simulink model "SquareRootEstimation"  (R2022b)
settings: Solver=ode23  StartTime=0.0  StopTime=10  RelTol=1e-7  AbsTol=1e-7
settings Model: Creator=aless  LastModifiedBy=aless

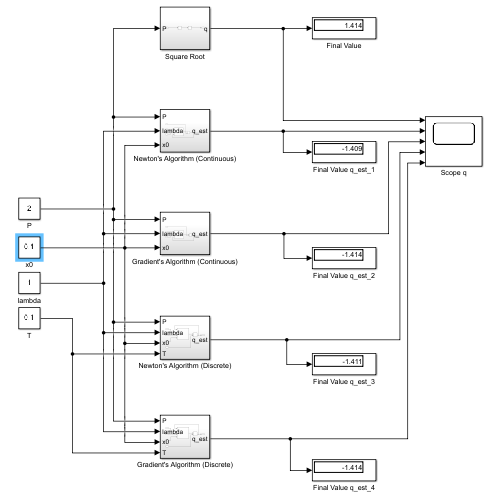
[thumbnail: Simulink's stored preview of the top-level diagram]
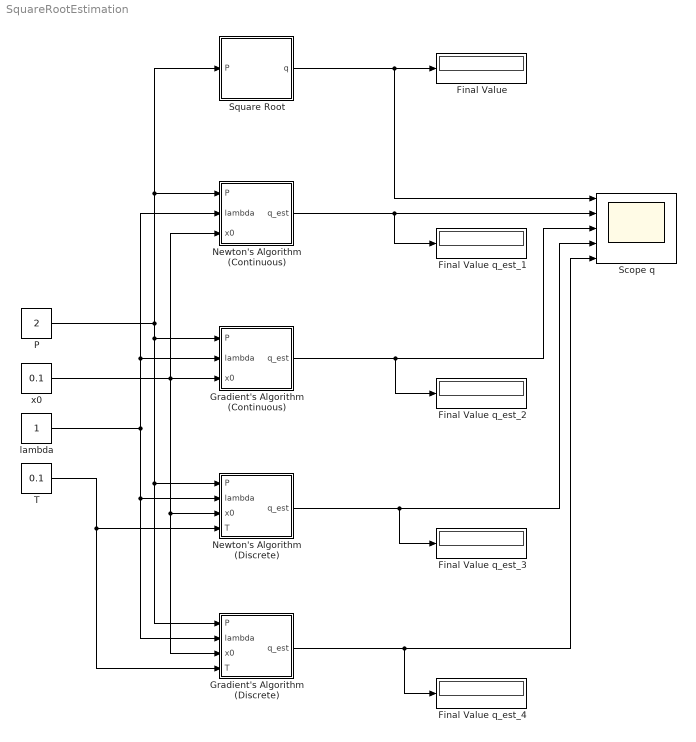
== system SquareRootEstimation ==
  Final Value : Display
  Final Value q_est_{1..4} (4 alike) : Display
  Gradient's Algorithm (Continuous) : Subsystem
  Gradient's Algorithm (Discrete) : Subsystem
  Newton's Algorithm (Continuous) : Subsystem
  Newton's Algorithm (Discrete) : Subsystem
  P : Constant  Value=2
  Scope q : Scope  NumInputPorts=5
  Square Root : Subsystem
  T : Constant  Value=0.1
  lambda : Constant
  x0 : Constant  Value=0.1
  wires:
  P/1 -> Square Root/1(P), Newton's Algorithm (Continuous)/1(P), Gradient's Algorithm (Discrete)/1(P), Newton's Algorithm (Discrete)/1(P), Gradient's Algorithm (Continuous)/1(P)
  lambda/1 -> Newton's Algorithm (Continuous)/2(lambda), Gradient's Algorithm (Continuous)/2(lambda), Gradient's Algorithm (Discrete)/2(lambda), Newton's Algorithm (Discrete)/2(lambda)
  Newton's Algorithm (Continuous)/1(q_est) -> Final Value q_est_1/1, Scope q/2
  Square Root/1(q) -> Scope q/1, Final Value/1
  Gradient's Algorithm (Continuous)/1(q_est) -> Final Value q_est_2/1, Scope q/3
  x0/1 -> Newton's Algorithm (Continuous)/3(x0), Gradient's Algorithm (Discrete)/3(x0), Newton's Algorithm (Discrete)/3(x0), Gradient's Algorithm (Continuous)/3(x0)
  Newton's Algorithm (Discrete)/1(q_est) -> Scope q/4, Final Value q_est_3/1
  Gradient's Algorithm (Discrete)/1(q_est) -> Final Value q_est_4/1, Scope q/5
  T/1 -> Gradient's Algorithm (Discrete)/4(T), Newton's Algorithm (Discrete)/4(T)

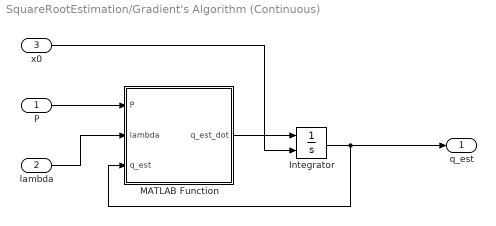
== system SquareRootEstimation/Gradient's Algorithm (Continuous) ==
  P : Inport
  lambda : Inport  Port=2
  x0 : Inport  Port=3
  Integrator : Integrator  InitialConditionSource=external  InitialCondition=0.1
  MATLAB Function : MATLAB Function  TreatAsAtomicUnit=on
  q_est : Outport
  wires:
  P/1 -> MATLAB Function/1(P)
  lambda/1 -> MATLAB Function/2(lambda)
  MATLAB Function/1(q_est_dot) -> Integrator/1
  Integrator/1 -> q_est/1, MATLAB Function/3(q_est)
  x0/1 -> Integrator/2

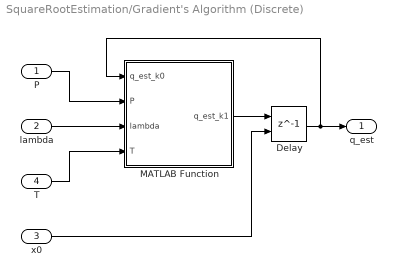
== system SquareRootEstimation/Gradient's Algorithm (Discrete) ==
  P : Inport
  lambda : Inport  Port=2
  x0 : Inport  Port=3
  T : Inport  Port=4
  Delay : Delay  DelayLength=1  InitialConditionSource=Input port  InitialCondition=0.1  SampleTime=0.1
      settings: InputPortMap=u0,p4
  MATLAB Function : MATLAB Function  TreatAsAtomicUnit=on
  q_est : Outport
  wires:
  P/1 -> MATLAB Function/2(P)
  lambda/1 -> MATLAB Function/3(lambda)
  T/1 -> MATLAB Function/4(T)
  MATLAB Function/1(q_est_k1) -> Delay/1
  Delay/1 -> MATLAB Function/1(q_est_k0), q_est/1
  x0/1 -> Delay/2

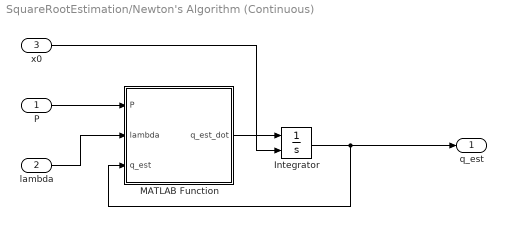
== system SquareRootEstimation/Newton's Algorithm (Continuous) ==
  P : Inport
  lambda : Inport  Port=2
  x0 : Inport  Port=3
  Integrator : Integrator  InitialConditionSource=external  InitialCondition=0.1
  MATLAB Function : MATLAB Function  TreatAsAtomicUnit=on
  q_est : Outport
  wires:
  P/1 -> MATLAB Function/1(P)
  lambda/1 -> MATLAB Function/2(lambda)
  MATLAB Function/1(q_est_dot) -> Integrator/1
  Integrator/1 -> q_est/1, MATLAB Function/3(q_est)
  x0/1 -> Integrator/2

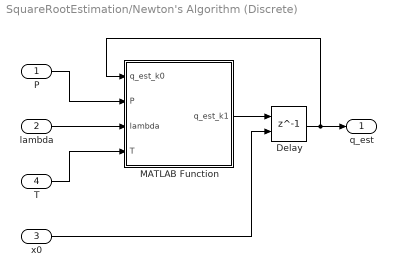
== system SquareRootEstimation/Newton's Algorithm (Discrete) ==
  P : Inport
  lambda : Inport  Port=2
  x0 : Inport  Port=3
  T : Inport  Port=4
  Delay : Delay  DelayLength=1  InitialConditionSource=Input port  InitialCondition=0.1  SampleTime=0.1
      settings: InputPortMap=u0,p4
  MATLAB Function : MATLAB Function  TreatAsAtomicUnit=on
  q_est : Outport
  wires:
  P/1 -> MATLAB Function/2(P)
  lambda/1 -> MATLAB Function/3(lambda)
  T/1 -> MATLAB Function/4(T)
  MATLAB Function/1(q_est_k1) -> Delay/1
  Delay/1 -> MATLAB Function/1(q_est_k0), q_est/1
  x0/1 -> Delay/2

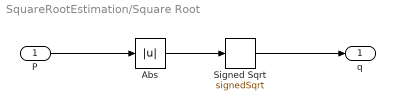
== system SquareRootEstimation/Square Root ==
  P : Inport
  Abs : Abs  SaturateOnIntegerOverflow=off
  Signed Sqrt : Sqrt  Operator=signedSqrt
  q : Outport
  wires:
  Abs/1 -> Signed Sqrt/1
  P/1 -> Abs/1
  Signed Sqrt/1 -> q/1

== matlab function SquareRootEstimation/Gradient's Algorithm (Continuous)/MATLAB Function ==
  data: P input; q_est_dot output; lambda input; q_est input
function q_est_dot = fcn(P, lambda, q_est)
jacobian = 2*q_est;
q_est_dot = lambda/2 * jacobian * (P - q_est*q_est);

== matlab function SquareRootEstimation/Newton's Algorithm (Continuous)/MATLAB Function ==
  data: P input; q_est_dot output; lambda input; q_est input
function q_est_dot = fcn(P, lambda, q_est)
jacobian = 2*q_est;
q_est_dot = lambda/2 * 1/jacobian * (P - q_est*q_est);

== matlab function SquareRootEstimation/Newton's Algorithm (Discrete)/MATLAB Function ==
  data: q_est_k0 input; P input; q_est_k1 output; lambda input; T input
function q_est_k1  = fcn(q_est_k0, P, lambda, T)

jacobian = 2*q_est_k0;
q_est_k1 = q_est_k0 + T*(lambda/2 * 1/jacobian * (P - q_est_k0*q_est_k0));

== matlab function SquareRootEstimation/Gradient's Algorithm (Discrete)/MATLAB Function ==
  data: q_est_k0 input; P input; q_est_k1 output; lambda input; T input
function q_est_k1  = fcn(q_est_k0, P, lambda, T)

jacobian = 2*q_est_k0;
q_est_k1 = q_est_k0 + T*(lambda/2 * jacobian * (P - q_est_k0*q_est_k0));
